simulink library "mbed_targets_stm_nucleo_f302r8"  (R2015a)
settings: Solver=ode45  StartTime=0.0  StopTime=10.0  RelTol=1e-3
libraries: mbed_lib x4
settings Model: CovSFcnEnable=off  Creator=oh  LastModifiedBy=oh
settings DebuggingCC: SolverPrmCheckMsg=warning

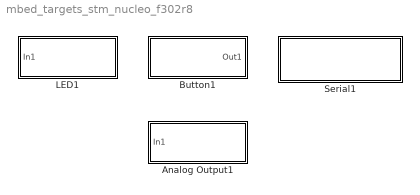
== system mbed_targets_stm_nucleo_f302r8 ==
  Analog Output1 : Subsystem  mask{Parameter1=0}
      mask Display:
      | offset=0.7;
      | plot([0+offset:0.025:0.25+offset],0.3*sin(2*pi*[0:0.1:1])+0.5)
      | port_label('input',1,['DAC1 (PA.4)']);
  Button1 : Subsystem  mask{Parameter1=0}
      mask Display:
      | plot([0 0.15 0.15 0.35 0.35 0.5],[0.3 0.3 0.7 0.7 0.3 0.3])
      | port_label('output',1,['UsrBtn1']);
  LED1 : Subsystem  mask{Parameter1=0}
      mask Display:
      | plot([0.5 0.65 0.65 0.85 0.85 1],[0.3 0.3 0.7 0.7 0.3 0.3])
      | port_label('input',1,['LED1']);
  Serial1 : Subsystem  mask{Parameter1=0, BaudRate=9600}
      mask prompts: BaudRate "Baud Rate:"
      mask TypeOptions BaudRate: Serial Configuration/BaudRate
      mask Display: disp(['Serial1(USB)\nTX:PA_2, RX:PA_3'])

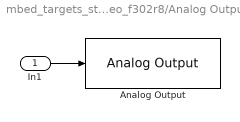
== system mbed_targets_stm_nucleo_f302r8/Analog Output1 ==
  In1 : Inport
  Analog Output : mbed_lib/GPIO/Analog Output  SParameter2=A  SParameter1=4  inputVariant=Double: 0 - 1.0f  SampleTime=-1
  wires:
  In1/1 -> Analog Output/1

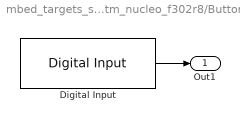
== system mbed_targets_stm_nucleo_f302r8/Button1 ==
  Digital Input : mbed_lib/GPIO/Digital Input  SParameter2=C  SParameter1=13  SParameter3=PullDefault  SampleTime=-1
  Out1 : Outport
  wires:
  Digital Input/1 -> Out1/1

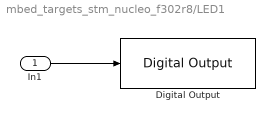
== system mbed_targets_stm_nucleo_f302r8/LED1 ==
  In1 : Inport
  Digital Output : mbed_lib/GPIO/Digital Output  SParameter2=B  SParameter1=13  SParameter3=PullDefault  SampleTime=-1
  wires:
  In1/1 -> Digital Output/1

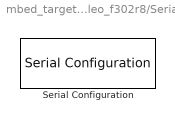
== system mbed_targets_stm_nucleo_f302r8/Serial1 ==
  Serial Configuration : mbed_lib/Serial/Serial Configuration  SerialPort=1  TXPort=A  TXPin=2  RXPort=A  RXPin=3  BaudRate=BaudRate
